simulink model "QCar2_lidar_point_cloud"  (R2023a)
settings: Solver=ode2  StartTime=0.0  StopTime=inf  FixedStep=1/20  RelTol=1e-3  EnableMultiTasking=on
undefined symbols (not defined in the file): gcbh, JPEG, Point, qc_get_step_size, video_display_show
libraries: quarc_library x10, simulink x1
settings Model: SimulationMode=external  ExtModeTrigDuration=10000  Creator=Quanser  LastModifiedBy=jpineros
settings SolverCC: AlgebraicLoopSolver=TrustRegion  PositivePriorityOrder=on
settings DataIOCC: ReturnWorkspaceOutputs=off
settings DebuggingCC: UnconnectedInputMsg=warning  UnconnectedOutputMsg=warning  UnconnectedLineMsg=warning  ArithmeticOperatorsInVariantConditions=warning
settings HardwareCC: ProdBitPerLong=64  ProdLargestAtomicInteger=LongLong  ProdLargestAtomicFloat=Double  ProdLongLongMode=on  ProdHWDeviceType=ARM Compatible->ARM 64-bit (LP64)
settings ModelReferenceCC: EnableRefExpFcnMdlSchedulingChecks=on
settings SFSimCC: CustomCodeUndefinedFunction=UseInterfaceOnly
settings RTWCC: Description=QUARC Linux QCar2 Target Using Toolchain  SystemTargetFile=quarc_linux_qcar2.tlc  TemplateMakefile=quarc_default_tmf  Toolchain=QUARC linux_qcar2 | gmake (64-bit Windows)  BuildConfiguration=Faster Runs
settings STFCustomTargetCC: SystemTargetFile=quarc_linux_qcar2.tlc
settings GRTTargetCC: ParMdlRefBuildCompliant=off  CompOptLevelCompliant=off  CombineOutputUpdateFcns=off  MatFileLogging=off  CPPClassGenCompliant=off  GRTInterface=on  ExtMode=on  ExtModeMexFile=quarc_comm  ExtModeMexArgs='-w -d /tmp -uri %u','tcpip://192.168.3.38:17001'
settings ConfigComp: CovBoundaryAbsTol=1.0e-5

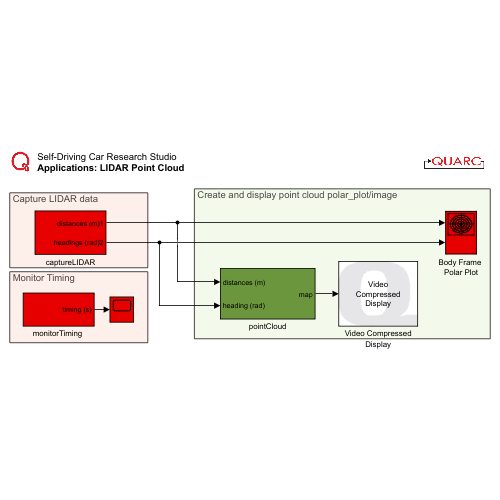
[thumbnail: Simulink's stored preview of the top-level diagram]
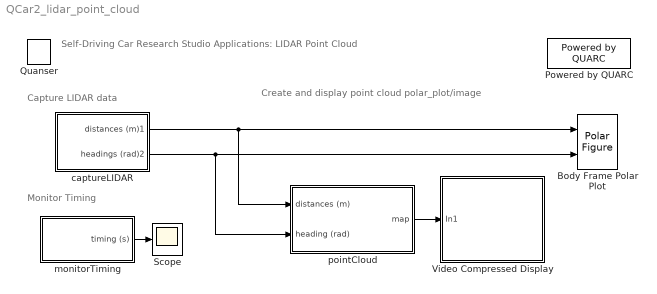
== system QCar2_lidar_point_cloud ==
  note: Monitor Timing
  note: Create and display point cloud polar_plot/image
  note: Capture LIDAR data
  note: Self-Driving Car Research Studio
      | Applications: LIDAR Point Cloud
  Body Frame Polar Plot : quarc_library/Sinks/Figures/Polar Figure  figure_mode=Use figure window  figure_tag=figure1  axes_tag=axes1  plot_mode=Frame-based  minimum_rho=0  maximum_rho=5  minimum_theta=0  maximum_theta=360  zero_location=top  direction=counterclockwise  buffer_size=1000  update_rate=1  sample_time=-1  initial_position="1.8          49.8         638.4         614.4"  initial_visibility=off  line1_style=None  line1_width=0.5  line1_color=[0 0.4470 0.7410]  marker1=Point (.)  marker1_size=1  marker1_edge_color=[0 0.447059 0.741176]  marker1_face_color=[0 0.447059 0.741176]  line2_style=Solid line (-)  line2_width=0.5  line2_color=[0.85098 0.32549 0.0980392]  marker2=None  marker2_size=6  marker2_edge_color=[0.85098 0.32549 0.0980392]  marker2_face_color=[0.85098 0.32549 0.0980392]  line3_style=Solid line (-)  line3_width=0.5  line3_color=[0.929412 0.694118 0.12549]  marker3=None  marker3_size=6  marker3_edge_color=[0.929412 0.694118 0.12549]  marker3_face_color=[0.929412 0.694118 0.12549]  line4_style=Solid line (-)  line4_width=0.5  line4_color=[0.494118 0.184314 0.556863]  marker4=None  marker4_size=6  marker4_edge_color=[0.494118 0.184314 0.556863]  marker4_face_color=[0.494118 0.184314 0.556863]  line5_style=Solid line (-)  line5_width=0.5  line5_color=[0.466667 0.67451 0.188235]  marker5=None  marker5_size=6  marker5_edge_color=[0.466667 0.67451 0.188235]  marker5_face_color=[0.466667 0.67451 0.188235]
      settings: SourceProductName=QUARC Targets
  Powered by QUARC : quarc_library/Logos/Powered by QUARC
  Quanser : quarc_library/Logos/Quanser
  Scope : Scope
  Video Compressed Display : Subsystem  LoadFcn=set_param(gcbh, 'UserData', gcb);  StartFcn=video_display_show([gcb, '/Video Display'], 'add', gcb);  mask(Video Compressed Display){algorithm=JPEG, quality=50, sample_time=-1, use_hardware=on}
      mask prompts: algorithm "Compression algorithm:"; quality "Compression quality (0-100):"; sample_time "Sample time (seconds):"; use_hardware "Use hardware acceleration for video display"
      mask help: Displays a video stream on the host, using compression to minimize bandwidth.
      mask init:
      | qc_set_display('Video\nCompressed\nDisplay');
      settings: UndoDeleteFcn=set_param(gcbh, 'UserData', gcb);  OpenFcn=video_display_show([gcb, '/Video Display'], 'show', gcb);  PreDeleteFcn=video_display_show([gcb, '/Video Display'], 'delete');
      settings: CopyFcn=|
      | set_param(gcbh, 'UserData', gcb);
      | set_param(gcbh, 'LinkStatus', 'none');
      settings: NameChangeFcn=|
      | video_display_show([get_param(gcbh, 'UserData'), '/Video Display'], 'rename', [gcb, '/Video Display']);
      | video_display_show([gcb, '/Video Display'], 'add', gcb);
      | set_param(gcbh, 'UserData', gcb);
      mask Help: web(qc_get_block_help_path(gcb));
      mask TypeOptions algorithm: Image Compress/algorithm
      mask TypeOptions quality: Image Compress/quality
      mask TypeOptions sample_time: Video Display/sample_time
      mask TypeOptions use_hardware: Video Display/use_hardware
      mask Display:
      | patch([0.98591 0.98591 0.62618 0.59072 0.56147   0.536   0.536  0.5441 0.56912 0.59207 0.60881 0.62276 0.63527 0.64364  0.6485  0.6485 0.64706 0.64499 0.63662 0.62411 0.61232 0.59837 0.58307 0.56147   0.536   0.536  0.5441  0.5747 0.60953 0.63662 0.67001  0.7034 0.72851 0.75425 0.77927 0.80294 0.82454 0.84119 0.85865 0.87395 0.88574 0.89339  0.8969 0.89969 0.89969 0.89267  0.8816 0.87044 0.85649  0.8384 0.81824 0.80294 0.78764 0.77513 0.76676 0.75776 0.76397 0.77513 0.79178 0.80987 0.82796 0.84326 0.86207 0.98528],[0.18689 0.05522 0.05522 0.05171 0.05171    0.05 0.18338 0.18338 0.19148 0.20435 0.22298 0.24863 0.28589 0.33125 0.38138 0.55139 0.59801 0.63761 0.68189 0.72149 0.74939 0.76694 0.77855 0.79367 0.79952 0.92768 0.92768 0.92768 0.92417 0.92066 0.91364  0.9032 0.89384 0.88106 0.86594 0.85073 0.82634 0.80537 0.77855 0.74363 0.70403 0.65858 0.61079 0.59099 0.41513 0.37202 0.31847 0.29048 0.25556 0.23342  0.2102 0.19382 0.18221 0.17285 0.16943 0.16124  0.1589 0.16241 0.16709 0.17168  0.1787 0.18221 0.18689 0.18689],[0.9,0.90,0.91])
      | patch([0.536 0.52601 0.46823 0.44528 0.41603 0.39101 0.35555 0.33116 0.31451 0.29291  0.2804 0.26717 0.25322 0.23999 0.22406 0.20732 0.19337 0.17528 0.15935 0.14396 0.13217 0.11759 0.10922 0.10085 0.09671 0.09392 0.09041 0.08906 0.08906 0.09464  0.0995 0.10778 0.11894 0.13145 0.14675 0.16349 0.17672 0.19409 0.20732 0.22406 0.23999 0.26159 0.27833 0.29849 0.31793 0.33602 0.35411 0.37085 0.39245 0.41603   0.536   0.536 0.53159 0.46409   0.446 0.42026 0.39587 0.37571 0.36113 0.34925 0.34088 0.33809 0.33809 0.34088 0.34583 0.35627 0.36392 0.38129 0.39587 0.41117 0.42719 0.44672  0.4676 0.48353 0.48353 0.52394   0.536],[0.05 0.04829 0.04712 0.04712 0.04829 0.05063 0.05405 0.05873 0.06107 0.06692 0.07043 0.07619 0.08087 0.08672 0.09482 0.10652 0.11696 0.13325  0.1508 0.17168 0.19499 0.22415 0.25439 0.28472 0.31379 0.35456 0.38489 0.41513 0.58055 0.63878 0.68774 0.72149 0.75641 0.78089 0.80537 0.82859 0.84029 0.85658 0.86594 0.87404  0.8834 0.89267 0.90086 0.90788 0.91247 0.91832 0.92066   0.923 0.92651 0.92768 0.92768 0.79952 0.79952 0.79952 0.79718 0.78899 0.77153 0.75056 0.72149 0.68072 0.62249  0.5549 0.41396 0.37085 0.33242 0.28121 0.25205 0.22181 0.20552 0.19499 0.18572 0.18221 0.17753 0.17636 0.17753  0.1787  0.1787],[0.9,0.90,0.91])
      | disp('Video\nCompressed\nDisplay');
  captureLIDAR : Subsystem
  "monitorTiming " : Subsystem
  pointCloud : Subsystem
  wires:
  captureLIDAR/1(distances (m)1) -> pointCloud/1(distances (m)), Body Frame Polar Plot/1
  captureLIDAR/2(headings (rad)2) -> pointCloud/2(heading (rad)), Body Frame Polar Plot/2
  "monitorTiming "/1(timing (s)) -> Scope/1
  pointCloud/1(map) -> Video Compressed Display/1(In1)

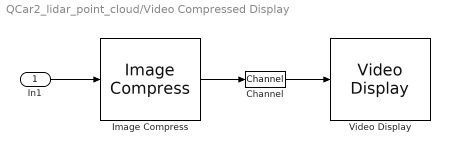
== system QCar2_lidar_point_cloud/Video Compressed Display ==
  In1 : Inport
  Channel : quarc_library/Signal Routing/Channel  channel=0  buffer_size=1
  Image Compress : quarc_library/Image Processing/Generic/Image Compress  algorithm=JPEG  source=Internal dialog parameter  quality=quality  output_dim=-1
  Video Display : quarc_library/Multimedia/Video Display  Tag=QCar2_lidar_point_cloud_/Video Compressed Display/Video Display  sample_time=sample_time  use_hardware=on
  wires:
  Image Compress/1 -> Channel/1
  In1/1 -> Image Compress/1
  Channel/1 -> Video Display/1

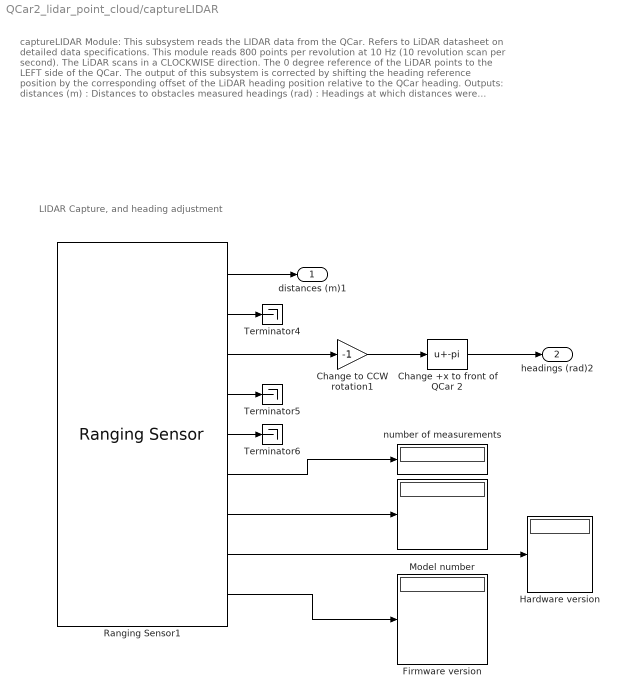
== system QCar2_lidar_point_cloud/captureLIDAR ==
  note: captureLIDAR Module:
      |
      | This subsystem reads the LIDAR data from the QCar. Refers to LiDAR datasheet on detailed data specifications.
      | This module reads 800 points per revolution at 10 Hz (10 revolution scan per second).
      | The LiDAR scans in a CLOCKWISE direction. The 0 degree reference of the LiDAR points to the LEFT side of the QCar.
      | The output of this subsystem is corrected by shifting the heading reference position by the corresponding offset of the LiDAR heading position relative to the QCar heading.
      |
      | Outputs:
      | distances (m) : Distances to obstacles measured
      | headings (rad) : Headings at which distances were measured (corrected relative to QCar heading)
  note: LIDAR Capture, and heading adjustment
  Change +x to front of QCar 2 : Bias  Bias=-pi  SaturateOnIntegerOverflow=off
  Change to CCW rotation1 : Gain  Gain=-1
  Firmware version : Display
  Hardware version : Display
  Model number : Display
  Ranging Sensor1 : quarc_library/Devices/Third-Party/Sensors/Ranging Sensor  sensor_type=RPLidar LIDAR  uri=serial-cpu://localhost:1?baud='256000',word='8',parity='none',stop='1',flow='none',dsr='on'  ranging_distance=Long  timing_budget=0.033  measurement_period=0.0005  output_mode=Fixed-size output  samples_per_revolution=1000  max_distance=0.050  max_angle=5  sample_time=qc_get_step_size  show_versions=on  active=on
      settings: SourceProductName=QUARC Targets
  Terminator4 : Terminator
  Terminator5 : Terminator
  Terminator6 : Terminator
  number of measurements : Display
  distances (m)1 : Outport  VectorParamsAs1DForOutWhenUnconnected=off
  headings (rad)2 : Outport  Port=2  VectorParamsAs1DForOutWhenUnconnected=off
  wires:
  Ranging Sensor1/6 -> number of measurements/1
  Ranging Sensor1/1 -> distances (m)1/1
  Ranging Sensor1/2 -> Terminator4/1
  Ranging Sensor1/5 -> Terminator6/1
  Ranging Sensor1/8 -> Hardware version/1
  Ranging Sensor1/7 -> Model number/1
  Ranging Sensor1/9 -> Firmware version/1
  Change to CCW rotation1/1 -> Change +x to front of QCar 2/1
  Ranging Sensor1/3 -> Change to CCW rotation1/1
  Change +x to front of QCar 2/1 -> headings (rad)2/1
  Ranging Sensor1/4 -> Terminator5/1

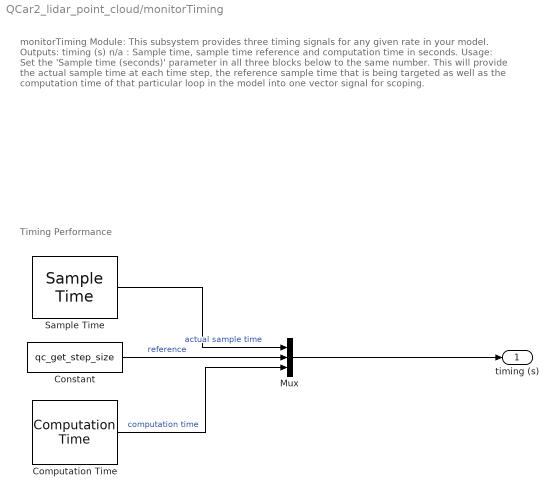
== system QCar2_lidar_point_cloud/monitorTiming  ==
  note: Timing Performance
  note: monitorTiming Module:
      |
      | This subsystem provides three timing signals for any given rate in your model.
      |
      | Outputs:
      | timing (s) n/a : Sample time, sample time reference and computation time in seconds.
      |
      | Usage:
      | Set the 'Sample time (seconds)' parameter in all three blocks below to the same number. This will provide the actual sample time at each time step, the reference sample time that is being targeted as well as the computation time of that particular loop in the model into one vector signal for scoping.
  Computation Time : quarc_library/Sources/Time/Computation Time  sample_time=qc_get_step_size  use_model=on  use_cpu_time=off
  Constant : Constant  Value=qc_get_step_size
  Mux : Mux  Inputs=3
  Sample Time : quarc_library/Sources/Time/Sample Time  Priority=-99  sample_time=qc_get_step_size
  timing (s) : Outport  VectorParamsAs1DForOutWhenUnconnected=off
  wires:
  Mux/1 -> timing (s)/1
  Computation Time/1 -> Mux/3  "computation time"
  Sample Time/1 -> Mux/1  "actual sample time"
  Constant/1 -> Mux/2  "reference"

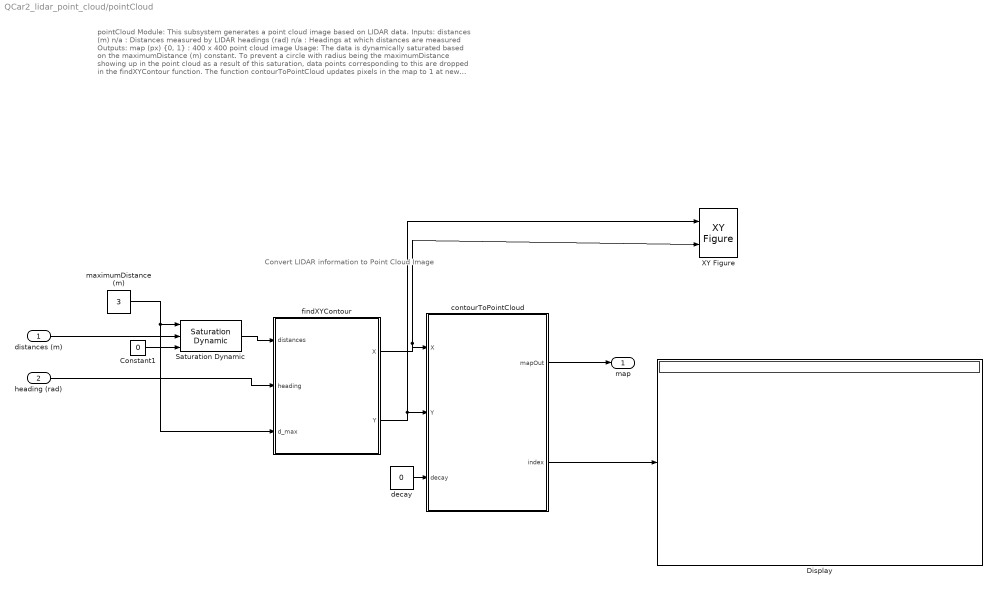
== system QCar2_lidar_point_cloud/pointCloud ==
  note: Convert LIDAR information to Point Cloud Image
  note: pointCloud Module:
      |
      | This subsystem generates a point cloud image based on LIDAR data.
      |
      | Inputs:
      | distances (m) n/a : Distances measured by LIDAR
      | headings (rad) n/a : Headings at which distances are measured
      |
      | Outputs:
      | map (px) {0, 1} : 400 x 400 point cloud image
      |
      | Usage:
      | The data is dynamically saturated based on the maximumDistance (m) constant. To prevent a circle with radius being the maximumDistance showing up in the point cloud as a result of this saturation, data points corresponding to this are dropped in the findXYContour function. The function contourToPointCloud updates pixels in the map to 1 at new locations, and decays older data at the rate specified by the decay parameter.
  distances (m) : Inport
  heading (rad) : Inport  Port=2
  Constant1 : Constant  Value=0
  Display : Display
  Saturation Dynamic : simulink/Discontinuities/Saturation Dynamic  OutMin=[]  OutMax=[]  OutDataTypeStr=Inherit: Same as second input  OutDataType=fixdt(1, 16)  OutScaling=2^-10  DoSatur=off
  XY Figure : quarc_library/Sinks/Figures/XY Figure  figure_mode=Use figure window  figure_tag=figure1  axes_tag=axes1  plot_mode=Frame-based  minimum_x=-3  maximum_x=3  minimum_y=-3  maximum_y=3  buffer_size=1000  update_rate=1  initial_position="641.8          49.8         638.4         614.4"  initial_visibility=off  sample_time=-1
      settings: SourceProductName=QUARC Targets
  contourToPointCloud : MATLAB Function  TreatAsAtomicUnit=on
  decay : Constant  Value=0
  findXYContour : MATLAB Function  TreatAsAtomicUnit=on
  maximumDistance (m) : Constant  Value=3
  map : Outport  VectorParamsAs1DForOutWhenUnconnected=off
  wires:
  distances (m)/1 -> Saturation Dynamic/2
  contourToPointCloud/1(mapOut) -> map/1
  Saturation Dynamic/1 -> findXYContour/1(distances)
  maximumDistance (m)/1 -> findXYContour/3(d_max), Saturation Dynamic/1
  Constant1/1 -> Saturation Dynamic/3
  decay/1 -> contourToPointCloud/3(decay)
  findXYContour/1(X) -> XY Figure/2, contourToPointCloud/1(X)
  findXYContour/2(Y) -> XY Figure/1, contourToPointCloud/2(Y)
  heading (rad)/1 -> findXYContour/2(heading)
  contourToPointCloud/2(index) -> Display/1

== matlab function QCar2_lidar_point_cloud/pointCloud/findXYContour ==
  data: distances input; X output size=1000; heading input; Y output size=1000; d_max input
function [X, Y] = findXYContour(distances, heading, d_max)

% find indices where distances corresponds to the d_max (bordering circle)
idx = distances < d_max;

% drop the bordering circle
temp_distances = distances(idx);
temp_heading = heading(idx);
% find X, Y pairs from distance, heading
X = temp_distances.*cos(temp_heading);
Y = temp_distances.*sin(temp_heading);

== matlab function QCar2_lidar_point_cloud/pointCloud/contourToPointCloud ==
  data: X input size=1000 [0..720]; mapOut output; Y input size=1000; decay input; index output
function [mapOut,index]= contourToPointCloud(X, Y, decay)

dim = 400; % Image size will be [dim x dim]
gain = 50; % 50 pixels per meter

persistent mapInternal
if isempty(mapInternal)
    mapInternal = zeros(dim, dim);
else
    mapInternal = decay*mapInternal; % decay older data... 
end

pX = round(dim/2 - X*gain); % X coordinates w.r.t image center
pY = round(dim/2 - Y*gain); % Y coordinates w.r.t image center

% At the locations corresponding to pX and pY, set a value of 1
% mapInternal(sub2ind([dim, dim], pX, pY)) = 1;
indexs=sub2ind([dim, dim], pX, pY);
index=indexs(1:1000);
mapInternal(index)=1;
mapOut = mapInternal;
